simulink model "Logic3"  (R2017a)
settings: Solver=VariableStepAuto  StartTime=0.0  StopTime=0.02  RelTol=1e-3
libraries: simulink x6
settings Model: Creator=VV  LastModifiedBy=mayartmal

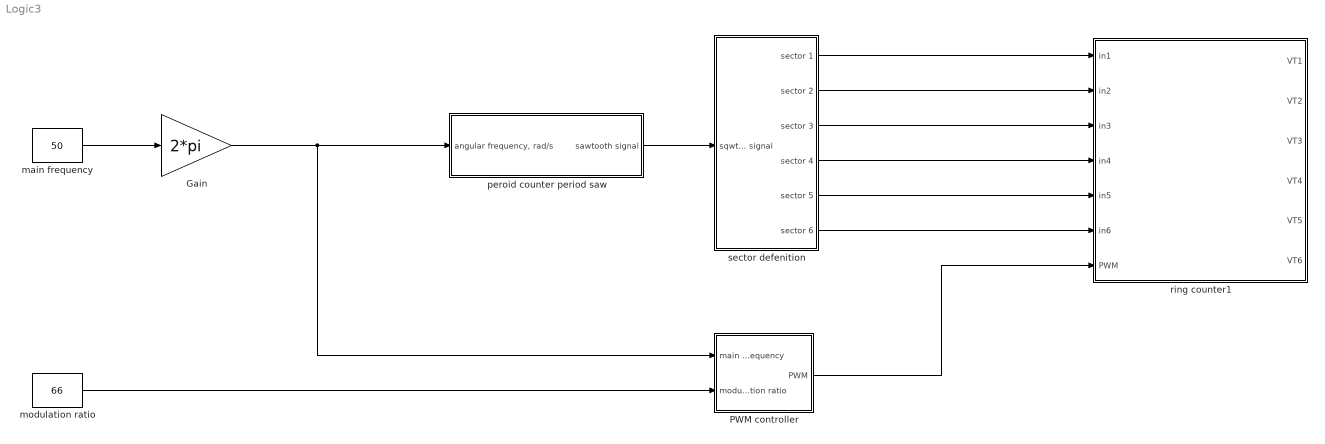
== system Logic3 ==
  Gain : Gain  Gain=2*pi
  PWM controller : Subsystem
  main frequency : Constant  Value=50  VectorParams1D=off  OutDataTypeStr=double
  modulation ratio : Constant  Value=66  VectorParams1D=off  OutDataTypeStr=double
  peroid counter period saw : Subsystem
  ring counter1 : MATLAB Function  TreatAsAtomicUnit=on
  sector defenition : Subsystem
  wires:
  main frequency/1 -> Gain/1
  Gain/1 -> PWM controller/1(main frequency), peroid counter period saw/1("angular frequency, rad/s")
  peroid counter period saw/1(sawtooth signal) -> sector defenition/1(sqwtooth signal)
  modulation ratio/1 -> PWM controller/2(modulation ratio)
  sector defenition/6(sector 6) -> ring counter1/6(in6)
  sector defenition/5(sector 5) -> ring counter1/5(in5)
  sector defenition/4(sector 4) -> ring counter1/4(in4)
  sector defenition/3(sector 3) -> ring counter1/3(in3)
  sector defenition/2(sector 2) -> ring counter1/2(in2)
  sector defenition/1(sector 1) -> ring counter1/1(in1)
  PWM controller/1(PWM) -> ring counter1/7(PWM)

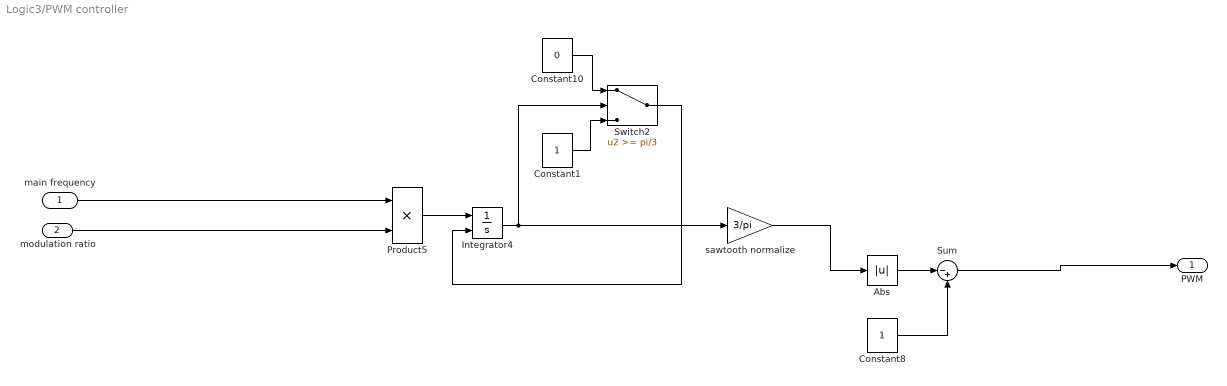
== system Logic3/PWM controller ==
  main frequency : Inport
  modulation ratio : Inport  Port=2
  Abs : Abs
  Constant1 : Constant  VectorParams1D=off  OutDataTypeStr=double
  Constant10 : Constant  Value=0  VectorParams1D=off  OutDataTypeStr=double
  Constant8 : Constant  VectorParams1D=off  OutDataTypeStr=double
  Integrator4 : Integrator  ExternalReset=falling  InitialCondition=-pi/3
  Product5 : Product
  Sum : Sum  Inputs=|-+
  Switch2 : Switch  Threshold=pi/3
  sawtooth normalize : Gain  Gain=3/pi
  PWM : Outport
  wires:
  main frequency/1 -> Product5/1
  Constant1/1 -> Switch2/3
  Constant8/1 -> Sum/2
  Abs/1 -> Sum/1
  Constant10/1 -> Switch2/1
  Integrator4/1 -> sawtooth normalize/1, Switch2/2
  Sum/1 -> PWM/1
  Switch2/1 -> Integrator4/2
  Product5/1 -> Integrator4/1
  sawtooth normalize/1 -> Abs/1
  modulation ratio/1 -> Product5/2

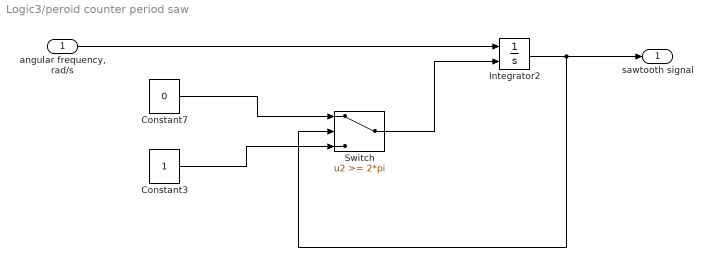
== system Logic3/peroid counter period saw ==
  "angular frequency, rad/s" : Inport
  Constant3 : Constant  VectorParams1D=off  OutDataTypeStr=double
  Constant7 : Constant  Value=0  VectorParams1D=off  OutDataTypeStr=double
  Integrator2 : Integrator  ExternalReset=falling
  Switch : Switch  Threshold=2*pi
  sawtooth signal : Outport
  wires:
  Constant7/1 -> Switch/1
  Switch/1 -> Integrator2/2
  Integrator2/1 -> sawtooth signal/1, Switch/2
  Constant3/1 -> Switch/3
  "angular frequency, rad/s"/1 -> Integrator2/1

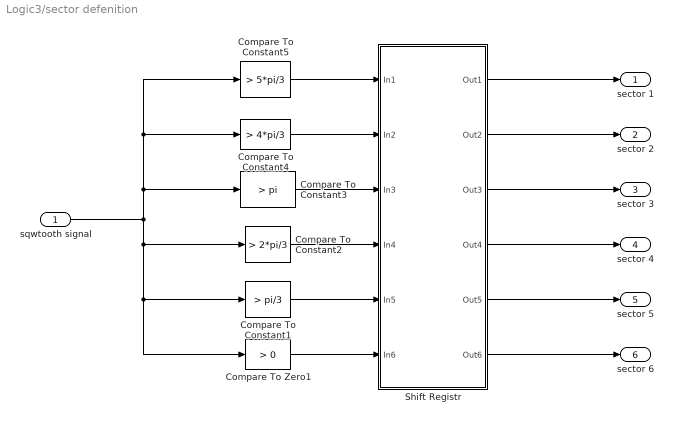
== system Logic3/sector defenition ==
  sqwtooth signal : Inport
  Compare To Constant1 : simulink/Logic and Bit Operations/Compare To Constant  relop=>  const=pi/3  OutDataTypeStr=boolean
  Compare To Constant2 : simulink/Logic and Bit Operations/Compare To Constant  relop=>  const=2*pi/3  OutDataTypeStr=boolean
  Compare To Constant3 : simulink/Logic and Bit Operations/Compare To Constant  relop=>  const=pi  OutDataTypeStr=boolean
  Compare To Constant4 : simulink/Logic and Bit Operations/Compare To Constant  relop=>  const=4*pi/3  OutDataTypeStr=boolean
  Compare To Constant5 : simulink/Logic and Bit Operations/Compare To Constant  relop=>  const=5*pi/3  OutDataTypeStr=boolean
  Compare To Zero1 : simulink/Logic and Bit Operations/Compare To Zero  relop=>  OutDataTypeStr=boolean
  Shift Registr : Subsystem
  sector 1 : Outport
  sector 2 : Outport  Port=2
  sector 3 : Outport  Port=3
  sector 4 : Outport  Port=4
  sector 5 : Outport  Port=5
  sector 6 : Outport  Port=6
  wires:
  Compare To Constant5/1 -> Shift Registr/1(In1)
  Compare To Constant4/1 -> Shift Registr/2(In2)
  Compare To Constant3/1 -> Shift Registr/3(In3)
  Compare To Constant2/1 -> Shift Registr/4(In4)
  Compare To Constant1/1 -> Shift Registr/5(In5)
  Compare To Zero1/1 -> Shift Registr/6(In6)
  Shift Registr/1(Out1) -> sector 1/1
  Shift Registr/2(Out2) -> sector 2/1
  Shift Registr/3(Out3) -> sector 3/1
  Shift Registr/4(Out4) -> sector 4/1
  Shift Registr/5(Out5) -> sector 5/1
  Shift Registr/6(Out6) -> sector 6/1
  sqwtooth signal/1 -> Compare To Zero1/1, Compare To Constant1/1, Compare To Constant2/1, Compare To Constant4/1, Compare To Constant5/1, Compare To Constant3/1

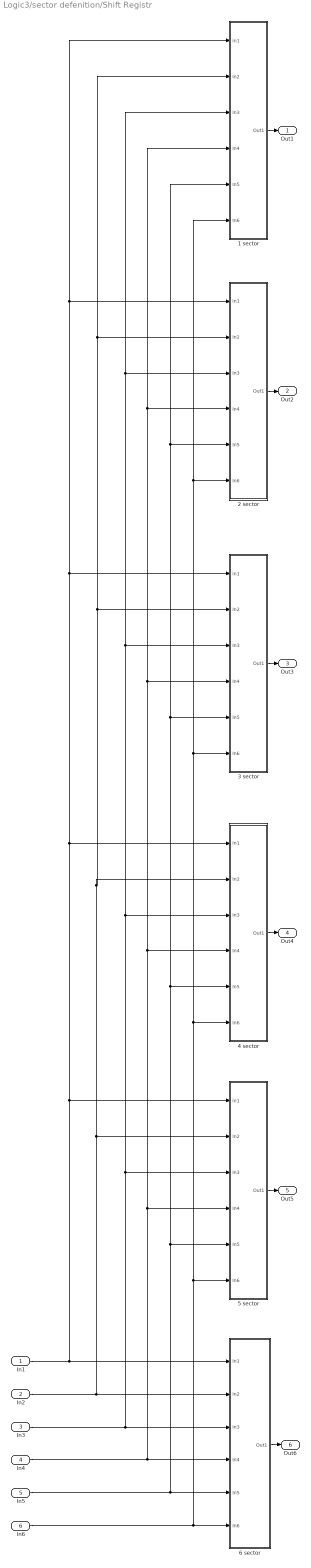
== system Logic3/sector defenition/Shift Registr ==
  In1 : Inport
  In2 : Inport  Port=2
  In3 : Inport  Port=3
  In4 : Inport  Port=4
  In5 : Inport  Port=5
  In6 : Inport  Port=6
  1 sector : Subsystem
  2 sector : Subsystem
  3 sector : Subsystem
  4 sector : Subsystem
  5 sector : Subsystem
  6 sector : Subsystem
  Out1 : Outport
  Out2 : Outport  Port=2
  Out3 : Outport  Port=3
  Out4 : Outport  Port=4
  Out5 : Outport  Port=5
  Out6 : Outport  Port=6
  wires:
  In6/1 -> 4 sector/6(In6), 1 sector/6(In6), 2 sector/6(In6), 3 sector/6(In6), 5 sector/6(In6), 6 sector/6(In6)
  In5/1 -> 3 sector/5(In5), 1 sector/5(In5), 2 sector/5(In5), 4 sector/5(In5), 5 sector/5(In5), 6 sector/5(In5)
  In4/1 -> 1 sector/4(In4), 2 sector/4(In4), 3 sector/4(In4), 4 sector/4(In4), 5 sector/4(In4), 6 sector/4(In4)
  In3/1 -> 4 sector/3(In3), 1 sector/3(In3), 2 sector/3(In3), 3 sector/3(In3), 5 sector/3(In3), 6 sector/3(In3)
  In2/1 -> 1 sector/2(In2), 2 sector/2(In2), 3 sector/2(In2), 4 sector/2(In2), 5 sector/2(In2), 6 sector/2(In2)
  In1/1 -> 1 sector/1(in1), 2 sector/1(in1), 3 sector/1(in1), 4 sector/1(in1), 5 sector/1(in1), 6 sector/1(In1)
  6 sector/1(Out1) -> Out6/1
  4 sector/1(Out1) -> Out4/1
  2 sector/1(Out1) -> Out2/1
  1 sector/1(Out1) -> Out1/1
  5 sector/1(Out1) -> Out5/1
  3 sector/1(Out1) -> Out3/1

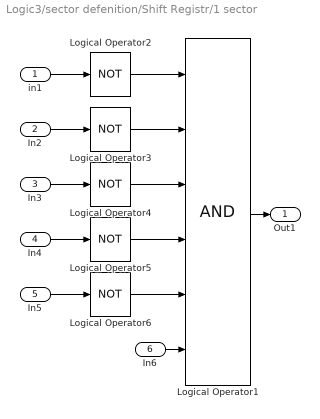
== system Logic3/sector defenition/Shift Registr/1 sector ==
  in1 : Inport
  In2 : Inport  Port=2
  In3 : Inport  Port=3
  In4 : Inport  Port=4
  In5 : Inport  Port=5
  In6 : Inport  Port=6
  Logical Operator1 : Logic  Inputs=6  AllPortsSameDT=off  OutDataTypeStr=boolean
  Logical Operator{2..6} (5 alike) : Logic  Operator=NOT  Inputs=6  AllPortsSameDT=off  OutDataTypeStr=boolean
  Out1 : Outport
  wires:
  Logical Operator5/1 -> Logical Operator1/4
  Logical Operator4/1 -> Logical Operator1/3
  Logical Operator3/1 -> Logical Operator1/2
  Logical Operator2/1 -> Logical Operator1/1
  in1/1 -> Logical Operator2/1
  In6/1 -> Logical Operator1/6
  In2/1 -> Logical Operator3/1
  Logical Operator1/1 -> Out1/1
  In5/1 -> Logical Operator6/1
  In3/1 -> Logical Operator4/1
  In4/1 -> Logical Operator5/1
  Logical Operator6/1 -> Logical Operator1/5

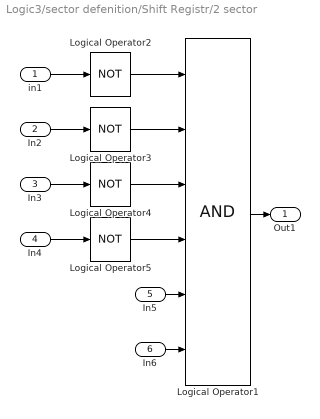
== system Logic3/sector defenition/Shift Registr/2 sector ==
  in1 : Inport
  In2 : Inport  Port=2
  In3 : Inport  Port=3
  In4 : Inport  Port=4
  In5 : Inport  Port=5
  In6 : Inport  Port=6
  Logical Operator1 : Logic  Inputs=6  AllPortsSameDT=off  OutDataTypeStr=boolean
  Logical Operator{2..5} (4 alike) : Logic  Operator=NOT  Inputs=6  AllPortsSameDT=off  OutDataTypeStr=boolean
  Out1 : Outport
  wires:
  In4/1 -> Logical Operator5/1
  In3/1 -> Logical Operator4/1
  In5/1 -> Logical Operator1/5
  Logical Operator1/1 -> Out1/1
  In2/1 -> Logical Operator3/1
  In6/1 -> Logical Operator1/6
  in1/1 -> Logical Operator2/1
  Logical Operator2/1 -> Logical Operator1/1
  Logical Operator3/1 -> Logical Operator1/2
  Logical Operator4/1 -> Logical Operator1/3
  Logical Operator5/1 -> Logical Operator1/4

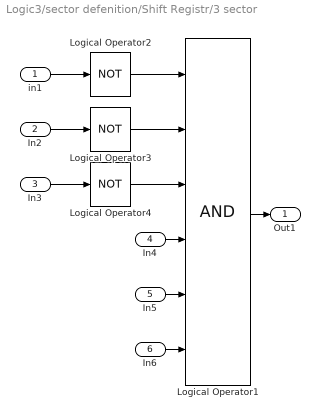
== system Logic3/sector defenition/Shift Registr/3 sector ==
  in1 : Inport
  In2 : Inport  Port=2
  In3 : Inport  Port=3
  In4 : Inport  Port=4
  In5 : Inport  Port=5
  In6 : Inport  Port=6
  Logical Operator1 : Logic  Inputs=6  AllPortsSameDT=off  OutDataTypeStr=boolean
  Logical Operator2 : Logic  Operator=NOT  Inputs=6  AllPortsSameDT=off  OutDataTypeStr=boolean
  Logical Operator3 : Logic  Operator=NOT  Inputs=6  AllPortsSameDT=off  OutDataTypeStr=boolean
  Logical Operator4 : Logic  Operator=NOT  Inputs=6  AllPortsSameDT=off  OutDataTypeStr=boolean
  Out1 : Outport
  wires:
  Logical Operator3/1 -> Logical Operator1/2
  Logical Operator2/1 -> Logical Operator1/1
  in1/1 -> Logical Operator2/1
  In6/1 -> Logical Operator1/6
  In2/1 -> Logical Operator3/1
  Logical Operator1/1 -> Out1/1
  In5/1 -> Logical Operator1/5
  In3/1 -> Logical Operator4/1
  In4/1 -> Logical Operator1/4
  Logical Operator4/1 -> Logical Operator1/3

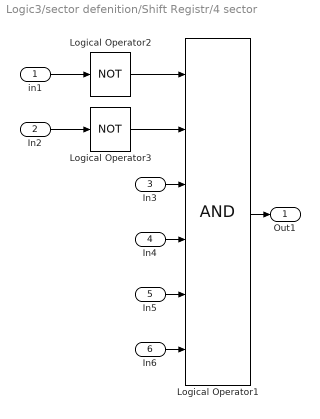
== system Logic3/sector defenition/Shift Registr/4 sector ==
  in1 : Inport
  In2 : Inport  Port=2
  In3 : Inport  Port=3
  In4 : Inport  Port=4
  In5 : Inport  Port=5
  In6 : Inport  Port=6
  Logical Operator1 : Logic  Inputs=6  AllPortsSameDT=off  OutDataTypeStr=boolean
  Logical Operator2 : Logic  Operator=NOT  Inputs=6  AllPortsSameDT=off  OutDataTypeStr=boolean
  Logical Operator3 : Logic  Operator=NOT  Inputs=6  AllPortsSameDT=off  OutDataTypeStr=boolean
  Out1 : Outport
  wires:
  In4/1 -> Logical Operator1/4
  In3/1 -> Logical Operator1/3
  In5/1 -> Logical Operator1/5
  Logical Operator1/1 -> Out1/1
  In2/1 -> Logical Operator3/1
  In6/1 -> Logical Operator1/6
  in1/1 -> Logical Operator2/1
  Logical Operator2/1 -> Logical Operator1/1
  Logical Operator3/1 -> Logical Operator1/2

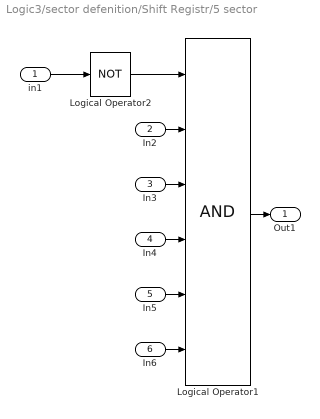
== system Logic3/sector defenition/Shift Registr/5 sector ==
  in1 : Inport
  In2 : Inport  Port=2
  In3 : Inport  Port=3
  In4 : Inport  Port=4
  In5 : Inport  Port=5
  In6 : Inport  Port=6
  Logical Operator1 : Logic  Inputs=6  AllPortsSameDT=off  OutDataTypeStr=boolean
  Logical Operator2 : Logic  Operator=NOT  Inputs=6  AllPortsSameDT=off  OutDataTypeStr=boolean
  Out1 : Outport
  wires:
  Logical Operator2/1 -> Logical Operator1/1
  in1/1 -> Logical Operator2/1
  In6/1 -> Logical Operator1/6
  In2/1 -> Logical Operator1/2
  Logical Operator1/1 -> Out1/1
  In5/1 -> Logical Operator1/5
  In3/1 -> Logical Operator1/3
  In4/1 -> Logical Operator1/4

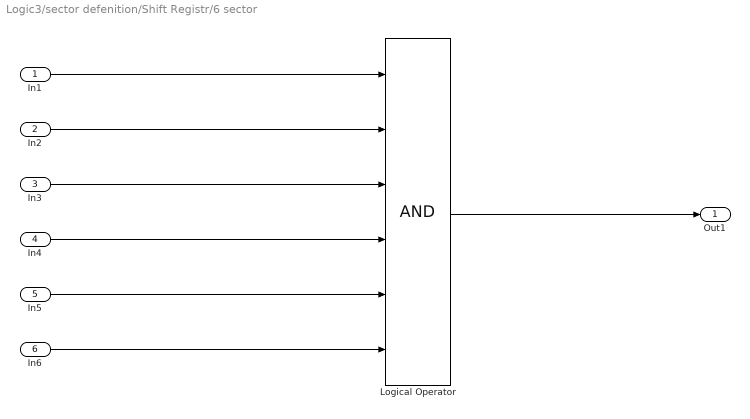
== system Logic3/sector defenition/Shift Registr/6 sector ==
  In1 : Inport
  In2 : Inport  Port=2
  In3 : Inport  Port=3
  In4 : Inport  Port=4
  In5 : Inport  Port=5
  In6 : Inport  Port=6
  Logical Operator : Logic  Inputs=6  AllPortsSameDT=off  OutDataTypeStr=boolean
  Out1 : Outport
  wires:
  Logical Operator/1 -> Out1/1
  In1/1 -> Logical Operator/1
  In4/1 -> Logical Operator/4
  In5/1 -> Logical Operator/5
  In6/1 -> Logical Operator/6
  In3/1 -> Logical Operator/3
  In2/1 -> Logical Operator/2

== matlab function Logic3/ring counter1 ==
  data: in1 input; in2 input; in3 input; in4 input; in5 input; in6 input; VT1 output; PWM input; VT2 output; VT3 output; VT4 output; VT5 output; VT6 output
function [VT1, VT2, VT3, VT4, VT5, VT6] = fcn(in1, in2, in3, in4, in5, in6, PWM)

VT1 = in1 | (in2 & PWM) | in3 |(in5 & (~PWM));
VT2 = (in2 & (~PWM)) | in4 | (in5 & PWM) | in6;

VT3 = in3 | (in4 & PWM) | in5 |(in1 & (~PWM));
VT4 = (in4 & (~PWM)) | in6 | (in1 & PWM) | in2;

VT5 = in5 | (in6 & PWM) | in1 |(in3 & (~PWM));
VT6 = (in6 & (~PWM)) | in2 | (in3 & PWM) | in4;



end
